simulink model "PID_robot_3d_base_movil"  (Simulink 7.5)
settings: Solver=ode45  StartTime=0.0  StopTime=50  RelTol=1e-3
libraries: simulink x3
settings Model: Creator=Patricio  LastModifiedBy=Patricio

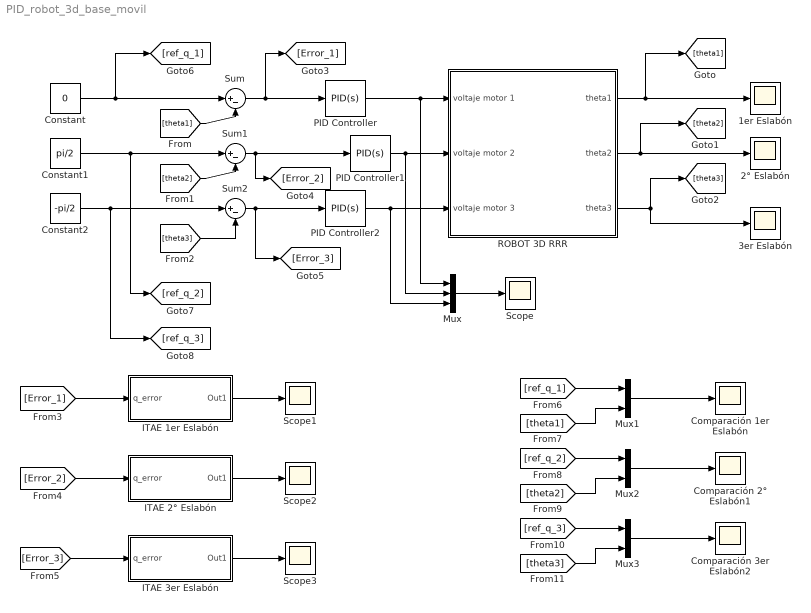
== system PID_robot_3d_base_movil ==
  1er Eslabón : Scope
      settings: TimeRange=5  YMin=-5000  YMax=-1750  MaxDataPoints=50000
  2° Eslabón : Scope
      settings: YMin=15.64  YMax=15.78  MaxDataPoints=50000
  3er Eslabón : Scope
      settings: TimeRange=30  YMin=-6.35  YMax=-6.21  SaveName=ScopeData2  MaxDataPoints=50000
  Comparación 1er Eslabón : Scope
      settings: TimeRange=30  YMin=-6.35  YMax=-6.21  SaveName=ScopeData10  MaxDataPoints=50000
  Comparación 2° Eslabón1 : Scope
      settings: TimeRange=30  YMin=-6.35  YMax=-6.21  SaveName=ScopeData8  MaxDataPoints=50000
  Comparación 3er Eslabón2 : Scope
      settings: TimeRange=30  YMin=-6.35  YMax=-6.21  SaveName=ScopeData18  MaxDataPoints=50000
  Constant : Constant  Value=0  OutDataType=fixdt(1, 16)  OutScaling=2^0
  Constant1 : Constant  Value=pi/2  OutDataType=fixdt(1, 16)  OutScaling=2^0
  Constant2 : Constant  Value=-pi/2  OutDataType=fixdt(1, 16)  OutScaling=2^0
  ITAE 1er Eslabón : Subsystem
  ITAE 2° Eslabón : Subsystem
  ITAE 3er Eslabón : Subsystem
  Mux : Mux  Inputs=3
  Mux1 : Mux  Inputs=2
  Mux2 : Mux  Inputs=2
  Mux3 : Mux  Inputs=2
  PID Controller : simulink/Continuous/PID Controller  DialogController=pidpack.PIDConfig.pidDDGCreate  DialogControllerArgs=DataTag0  SystemSampleTime=-1  Controller=PID  TimeDomain=Continuous-time  SampleTime=1  IntegratorMethod=Forward Euler  FilterMethod=Forward Euler  Form=Parallel  P=10  I=0  D=1  N=100  InitialConditionSource=internal  InitialConditionForIntegrator=0  InitialConditionForFilter=0  ExternalReset=none  LimitOutput=off  UpperSaturationLimit=inf  LowerSaturationLimit=-inf  LinearizeAsGain=off  AntiWindupMode=none  Kb=1  TrackingMode=off  Kt=1  PParamMin=[]  PParamMax=[]  IParamMin=[]  IParamMax=[]  DParamMin=[]  DParamMax=[]  NParamMin=[]  NParamMax=[]  KbParamMin=[]  KbParamMax=[]  KtParamMin=[]  KtParamMax=[]  POutMin=[]  POutMax=[]  IOutMin=[]  IOutMax=[]  DOutMin=[]  DOutMax=[]  NOutMin=[]  NOutMax=[]  KbOutMin=[]  KbOutMax=[]  KtOutMin=[]  KtOutMax=[]  IntegratorOutMin=[]  IntegratorOutMax=[]  FilterOutMin=[]  FilterOutMax=[]  SumOutMin=[]  SumOutMax=[]  SumI1OutMin=[]  SumI1OutMax=[]  SumI2OutMin=[]  SumI2OutMax=[]  SumI3OutMin=[]  SumI3OutMax=[]  SumDOutMin=[]  SumDOutMax=[]  SaturationOutMin=[]  SaturationOutMax=[]  IntegratorContinuousStateAttributes=''  IntegratorStateMustResolveToSignalObject=off  IntegratorRTWStateStorageClass=Auto  FilterContinuousStateAttributes=''  FilterStateMustResolveToSignalObject=off  FilterRTWStateStorageClass=Auto
  PID Controller1 : simulink/Continuous/PID Controller  DialogController=pidpack.PIDConfig.pidDDGCreate  DialogControllerArgs=DataTag1  SystemSampleTime=-1  Controller=PID  TimeDomain=Continuous-time  SampleTime=1  IntegratorMethod=Forward Euler  FilterMethod=Forward Euler  Form=Parallel  P=10  I=2  D=1  N=100  InitialConditionSource=internal  InitialConditionForIntegrator=0  InitialConditionForFilter=0  ExternalReset=none  LimitOutput=off  UpperSaturationLimit=inf  LowerSaturationLimit=-inf  LinearizeAsGain=off  AntiWindupMode=none  Kb=1  TrackingMode=off  Kt=1  PParamMin=[]  PParamMax=[]  IParamMin=[]  IParamMax=[]  DParamMin=[]  DParamMax=[]  NParamMin=[]  NParamMax=[]  KbParamMin=[]  KbParamMax=[]  KtParamMin=[]  KtParamMax=[]  POutMin=[]  POutMax=[]  IOutMin=[]  IOutMax=[]  DOutMin=[]  DOutMax=[]  NOutMin=[]  NOutMax=[]  KbOutMin=[]  KbOutMax=[]  KtOutMin=[]  KtOutMax=[]  IntegratorOutMin=[]  IntegratorOutMax=[]  FilterOutMin=[]  FilterOutMax=[]  SumOutMin=[]  SumOutMax=[]  SumI1OutMin=[]  SumI1OutMax=[]  SumI2OutMin=[]  SumI2OutMax=[]  SumI3OutMin=[]  SumI3OutMax=[]  SumDOutMin=[]  SumDOutMax=[]  SaturationOutMin=[]  SaturationOutMax=[]  IntegratorContinuousStateAttributes=''  IntegratorStateMustResolveToSignalObject=off  IntegratorRTWStateStorageClass=Auto  FilterContinuousStateAttributes=''  FilterStateMustResolveToSignalObject=off  FilterRTWStateStorageClass=Auto
  PID Controller2 : simulink/Continuous/PID Controller  DialogController=pidpack.PIDConfig.pidDDGCreate  DialogControllerArgs=DataTag2  SystemSampleTime=-1  Controller=PID  TimeDomain=Continuous-time  SampleTime=1  IntegratorMethod=Forward Euler  FilterMethod=Forward Euler  Form=Parallel  P=10  I=0  D=1  N=100  InitialConditionSource=internal  InitialConditionForIntegrator=0  InitialConditionForFilter=0  ExternalReset=none  LimitOutput=off  UpperSaturationLimit=inf  LowerSaturationLimit=-inf  LinearizeAsGain=off  AntiWindupMode=none  Kb=1  TrackingMode=off  Kt=1  PParamMin=[]  PParamMax=[]  IParamMin=[]  IParamMax=[]  DParamMin=[]  DParamMax=[]  NParamMin=[]  NParamMax=[]  KbParamMin=[]  KbParamMax=[]  KtParamMin=[]  KtParamMax=[]  POutMin=[]  POutMax=[]  IOutMin=[]  IOutMax=[]  DOutMin=[]  DOutMax=[]  NOutMin=[]  NOutMax=[]  KbOutMin=[]  KbOutMax=[]  KtOutMin=[]  KtOutMax=[]  IntegratorOutMin=[]  IntegratorOutMax=[]  FilterOutMin=[]  FilterOutMax=[]  SumOutMin=[]  SumOutMax=[]  SumI1OutMin=[]  SumI1OutMax=[]  SumI2OutMin=[]  SumI2OutMax=[]  SumI3OutMin=[]  SumI3OutMax=[]  SumDOutMin=[]  SumDOutMax=[]  SaturationOutMin=[]  SaturationOutMax=[]  IntegratorContinuousStateAttributes=''  IntegratorStateMustResolveToSignalObject=off  IntegratorRTWStateStorageClass=Auto  FilterContinuousStateAttributes=''  FilterStateMustResolveToSignalObject=off  FilterRTWStateStorageClass=Auto
  ROBOT 3D RRR : Subsystem
  Scope{,1..3} (4 alike) : Scope
      Scope settings: SaveName=ScopeData9
      Scope1 settings: SaveName=ScopeData15
      Scope2 settings: SaveName=ScopeData16
      Scope3 settings: SaveName=ScopeData17
  Sum : Sum  Inputs=|+-  OutDataType=fixdt(1, 16)  OutScaling=2^0
  Sum1 : Sum  Inputs=|+-  OutDataType=fixdt(1, 16)  OutScaling=2^0
  Sum2 : Sum  Inputs=|+-  OutDataType=fixdt(1, 16)  OutScaling=2^0
  wires:
  Sum/1 -> PID Controller/1, [Error_1]
  ROBOT 3D RRR/1(theta1) -> 1er Eslabón/1, [theta1]
  ROBOT 3D RRR/2(theta2) -> 2° Eslabón/1, [theta2]
  ROBOT 3D RRR/3(theta3) -> 3er Eslabón/1, [theta3]
  [theta1] -> Sum/2
  Sum1/1 -> PID Controller1/1, [Error_2]
  Sum2/1 -> PID Controller2/1, [Error_3]
  [theta2] -> Sum1/2
  [theta3] -> Sum2/2
  PID Controller/1 -> ROBOT 3D RRR/1(voltaje motor 1), Mux/1
  PID Controller1/1 -> ROBOT 3D RRR/2(voltaje motor 2), Mux/2
  PID Controller2/1 -> ROBOT 3D RRR/3(voltaje motor 3), Mux/3
  Mux/1 -> Scope/1
  Mux1/1 -> Comparación 1er Eslabón/1
  Constant2/1 -> Sum2/1, [ref_q_3]
  Constant1/1 -> Sum1/1, [ref_q_2]
  Constant/1 -> Sum/1, [ref_q_1]
  ITAE 1er Eslabón/1(Out1) -> Scope1/1
  ITAE 2° Eslabón/1(Out1) -> Scope2/1
  ITAE 3er Eslabón/1(Out1) -> Scope3/1
  [Error_1] -> ITAE 1er Eslabón/1(q_error)
  [Error_2] -> ITAE 2° Eslabón/1(q_error)
  [Error_3] -> ITAE 3er Eslabón/1(q_error)
  [ref_q_1] -> Mux1/1
  [theta1] -> Mux1/2
  Mux2/1 -> Comparación 2° Eslabón1/1
  [ref_q_2] -> Mux2/1
  [theta2] -> Mux2/2
  Mux3/1 -> Comparación 3er Eslabón2/1
  [ref_q_3] -> Mux3/1
  [theta3] -> Mux3/2

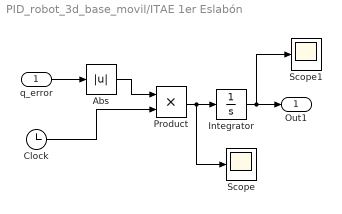
== system PID_robot_3d_base_movil/ITAE 1er Eslabón ==
  q_error : Inport  OutDataType=fixdt(1, 16)  OutScaling=2^0
  Abs : Abs  OutDataType=fixdt(1, 16)  OutScaling=2^0
  Clock : Clock
      settings: Decimation=10
  Integrator : Integrator
  Product : Product  OutDataType=fixdt(1, 16)  OutScaling=2^0  RndMeth=Zero
  Scope : Scope
      settings: SaveName=ScopeData6
  Scope1 : Scope
      settings: SaveName=ScopeData7
  Out1 : Outport  OutDataType=fixdt(1, 16)  OutScaling=2^0
  wires:
  q_error/1 -> Abs/1
  Abs/1 -> Product/1
  Clock/1 -> Product/2
  Product/1 -> Integrator/1, Scope/1
  Integrator/1 -> Out1/1, Scope1/1

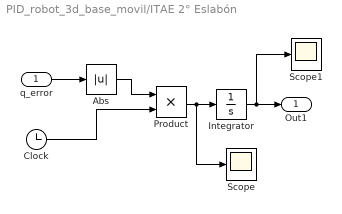
== system PID_robot_3d_base_movil/ITAE 2° Eslabón ==
  q_error : Inport  OutDataType=fixdt(1, 16)  OutScaling=2^0
  Abs : Abs  OutDataType=fixdt(1, 16)  OutScaling=2^0
  Clock : Clock
      settings: Decimation=10
  Integrator : Integrator
  Product : Product  OutDataType=fixdt(1, 16)  OutScaling=2^0  RndMeth=Zero
  Scope : Scope
      settings: SaveName=ScopeData6
  Scope1 : Scope
      settings: SaveName=ScopeData7
  Out1 : Outport  OutDataType=fixdt(1, 16)  OutScaling=2^0
  wires:
  Integrator/1 -> Scope1/1, Out1/1
  Product/1 -> Scope/1, Integrator/1
  Clock/1 -> Product/2
  Abs/1 -> Product/1
  q_error/1 -> Abs/1

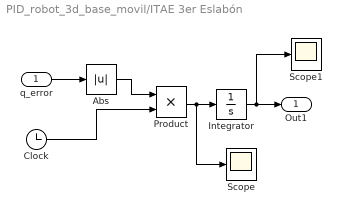
== system PID_robot_3d_base_movil/ITAE 3er Eslabón ==
  q_error : Inport  OutDataType=fixdt(1, 16)  OutScaling=2^0
  Abs : Abs  OutDataType=fixdt(1, 16)  OutScaling=2^0
  Clock : Clock
      settings: Decimation=10
  Integrator : Integrator
  Product : Product  OutDataType=fixdt(1, 16)  OutScaling=2^0  RndMeth=Zero
  Scope : Scope
      settings: SaveName=ScopeData6
  Scope1 : Scope
      settings: SaveName=ScopeData7
  Out1 : Outport  OutDataType=fixdt(1, 16)  OutScaling=2^0
  wires:
  q_error/1 -> Abs/1
  Abs/1 -> Product/1
  Clock/1 -> Product/2
  Product/1 -> Integrator/1, Scope/1
  Integrator/1 -> Out1/1, Scope1/1

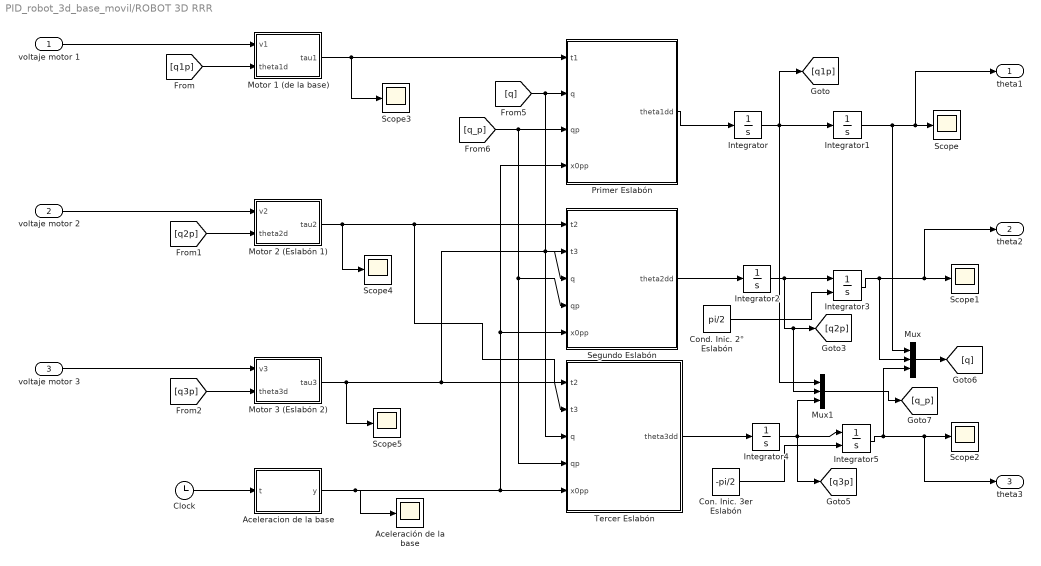
== system PID_robot_3d_base_movil/ROBOT 3D RRR ==
  voltaje motor 1 : Inport  OutDataType=fixdt(1, 16)  OutScaling=2^0
  voltaje motor 2 : Inport  Port=2  OutDataType=fixdt(1, 16)  OutScaling=2^0
  voltaje motor 3 : Inport  Port=3  OutDataType=fixdt(1, 16)  OutScaling=2^0
  Aceleracion de la base : Stateflow chart  TreatAsAtomicUnit=on
  Aceleración de la base : Scope
      settings: SaveName=ScopeData14  MaxDataPoints=50000
  Clock : Clock
      settings: Decimation=10
  Con. Inic. 3er Eslabón : Constant  Value=-pi/2  OutDataType=fixdt(1, 16)  OutScaling=2^0
  Cond. Inic. 2° Eslabón : Constant  Value=pi/2  OutDataType=fixdt(1, 16)  OutScaling=2^0
  Integrator{,1..2,4} (4 alike) : Integrator
  Integrator3 : Integrator  InitialConditionSource=external  InitialCondition=-pi/2
  Integrator5 : Integrator  InitialConditionSource=external
  Motor 1 (de la base) : Stateflow chart  TreatAsAtomicUnit=on
  Motor 2 (Eslabón 1) : Stateflow chart  TreatAsAtomicUnit=on
  Motor 3 (Eslabón 2) : Stateflow chart  TreatAsAtomicUnit=on
  Mux : Mux  Inputs=3
  Mux1 : Mux  Inputs=3
  Primer Eslabón : Stateflow chart  TreatAsAtomicUnit=on
      settings: MinAlgLoopOccurrences=on
  Scope{,1..5} (6 alike) : Scope
      Scope settings: SaveName=ScopeData3
      Scope1 settings: SaveName=ScopeData4
      Scope2 settings: SaveName=ScopeData5
      Scope3 settings: SaveName=ScopeData11
      Scope4 settings: SaveName=ScopeData12
      Scope5 settings: SaveName=ScopeData13
  Segundo Eslabón : Stateflow chart  TreatAsAtomicUnit=on
      settings: MinAlgLoopOccurrences=on
  Tercer Eslabón : Stateflow chart  TreatAsAtomicUnit=on
      settings: MinAlgLoopOccurrences=on
  theta1 : Outport  OutDataType=fixdt(1, 16)  OutScaling=2^0
  theta2 : Outport  Port=2  OutDataType=fixdt(1, 16)  OutScaling=2^0
  theta3 : Outport  Port=3  OutDataType=fixdt(1, 16)  OutScaling=2^0
  wires:
  Integrator/1 -> Integrator1/1, Mux1/1, [q1p]
  Primer Eslabón/1(theta1dd) -> Integrator/1
  Motor 1 (de la base)/1(tau1) -> Primer Eslabón/1(t1), Scope3/1
  [q] -> Primer Eslabón/2(q), Segundo Eslabón/3(q), Tercer Eslabón/3(q)
  [q_p] -> Primer Eslabón/3(qp), Segundo Eslabón/4(qp), Tercer Eslabón/4(qp)
  [q1p] -> Motor 1 (de la base)/2(theta1d)
  Motor 2 (Eslabón 1)/1(tau2) -> Scope4/1, Segundo Eslabón/1(t2), Tercer Eslabón/1(t2)
  [q2p] -> Motor 2 (Eslabón 1)/2(theta2d)
  Integrator2/1 -> Integrator3/1, [q2p], Mux1/2
  Integrator3/1 -> Mux/2, Scope1/1, theta2/1
  Motor 3 (Eslabón 2)/1(tau3) -> Scope5/1, Tercer Eslabón/2(t3), Segundo Eslabón/2(t3)
  Tercer Eslabón/1(theta3dd) -> Integrator4/1
  Integrator4/1 -> Integrator5/1, [q3p], Mux1/3
  Integrator5/1 -> Mux/3, Scope2/1, theta3/1
  [q3p] -> Motor 3 (Eslabón 2)/2(theta3d)
  Mux/1 -> [q]
  Mux1/1 -> [q_p]
  Segundo Eslabón/1(theta2dd) -> Integrator2/1
  Integrator1/1 -> Mux/1, Scope/1, theta1/1
  Cond. Inic. 2° Eslabón/1 -> Integrator3/2
  Con. Inic. 3er Eslabón/1 -> Integrator5/2
  Clock/1 -> Aceleracion de la base/1(t)
  Aceleracion de la base/1(y) -> Aceleración de la base/1, Tercer Eslabón/5(x0pp), Segundo Eslabón/5(x0pp), Primer Eslabón/4(x0pp)
  voltaje motor 3/1 -> Motor 3 (Eslabón 2)/1(v3)
  voltaje motor 2/1 -> Motor 2 (Eslabón 1)/1(v2)
  voltaje motor 1/1 -> Motor 1 (de la base)/1(v1)

== matlab function ROBOT 3D RRR/Aceleracion de la base ==
  data: t input double; y output double
function y = fcn(t)
%#eml
if t>=0 && t<2
    y=0;
elseif t>=2 && t<4
    y=0.5;
elseif t>=4 && t<6
    y=0;
elseif t>=6 && t<8
    y=-0.5;
else
    y=0;
end

== matlab function ROBOT 3D RRR/Motor 1 (de la base) ==
  data: v1 input double; tau1 output double; theta1d input double
function tau1 = fcn(v1,theta1d)
%#eml
%Voltaje entre 0 y 24 volts
N_1=50;
Kt=3; %en [volt/rad/seg]
Bm=0.1; %Roce viscozo [N.m/rad/seg]
R1=1;
tau1=(N_1*Kt*(v1/R1))-(Bm*theta1d);

== matlab function ROBOT 3D RRR/Primer Eslabón ==
  data: t1 input double; theta1dd output double; q input double size=3; qp input double size=3; x0pp input double
function theta1dd = fcn(t1,q,qp,x0pp)

theta1=q(1);
theta2=q(2);
theta3=q(3);

theta1d=qp(1);
theta2d=qp(2);
theta3d=qp(3);

a1=0.2;
a2=1;
a3=1;
b1=0.01;
%b2=0.01;
%b3=0.01;
%g=9.81;
m1=0.2;
m2=1;
m3=1;


theta1dd = (6*t1 - 6*b1*theta1d + 6*a1*m1*x0pp*sin(theta1) + 6*a1*m2*x0pp*sin(theta1) + 6*a1*m3*x0pp*sin(theta1) + 3*a2*m2*x0pp*cos(theta2)*sin(theta1) + 6*a2*m3*x0pp*cos(theta2)*sin(theta1) + 4*a2^2*m2*theta1d*theta2d*cos(theta2)*sin(theta2) + 12*a2^2*m3*theta1d*theta2d*cos(theta2)*sin(theta2) - 4*a3^2*m3*theta1d*theta2d*cos(theta2)*sin(theta2) - 4*a3^2*m3*theta1d*theta3d*cos(theta2)*sin(theta2) - 4*a3^2*m3*theta1d*theta2d*cos(theta3)*sin(theta3) - 4*a3^2*m3*theta1d*theta3d*cos(theta3)*sin(theta3) + 3*a3*m3*x0pp*cos(theta2)*cos(theta3)*sin(theta1) - 3*a3*m3*x0pp*sin(theta1)*sin(theta2)*sin(theta3) + 6*a1*a2*m2*theta1d*theta2d*sin(theta2) + 12*a1*a2*m3*theta1d*theta2d*sin(theta2) - 6*a2*a3*m3*theta1d*theta2d*sin(theta3) + 6*a1*a3*m3*theta1d*theta2d*cos(theta2)*sin(theta3) + 6*a1*a3*m3*theta1d*theta2d*cos(theta3)*sin(theta2) + 6*a1*a3*m3*theta1d*theta3d*cos(theta2)*sin(theta3) + 6*a1*a3*m3*theta1d*theta3d*cos(theta3)*sin(theta2) + 8*a3^2*m3*theta1d*theta2d*cos(theta2)*cos(theta3)^2*sin(theta2) + 8*a3^2*m3*theta1d*theta2d*cos(theta2)^2*cos(theta3)*sin(theta3) + 8*a3^2*m3*theta1d*theta3d*cos(theta2)*cos(theta3)^2*sin(theta2) + 8*a3^2*m3*theta1d*theta3d*cos(theta2)^2*cos(theta3)*sin(theta3) + 12*a2*a3*m3*theta1d*theta2d*cos(theta2)^2*sin(theta3) + 6*a2*a3*m3*theta1d*theta3d*cos(theta2)^2*sin(theta3) + 12*a2*a3*m3*theta1d*theta2d*cos(theta2)*cos(theta3)*sin(theta2) + 6*a2*a3*m3*theta1d*theta3d*cos(theta2)*cos(theta3)*sin(theta2))/(6*a1^2*m1 + 6*a1^2*m2 + 6*a1^2*m3 + 2*a3^2*m3 + 2*a2^2*m2*cos(theta2)^2 + 6*a2^2*m3*cos(theta2)^2 - 2*a3^2*m3*cos(theta2)^2 - 2*a3^2*m3*cos(theta3)^2 + 6*a1*a2*m2*cos(theta2) + 12*a1*a2*m3*cos(theta2) + 4*a3^2*m3*cos(theta2)^2*cos(theta3)^2 + 6*a1*a3*m3*cos(theta2)*cos(theta3) - 6*a1*a3*m3*sin(theta2)*sin(theta3) + 6*a2*a3*m3*cos(theta2)^2*cos(theta3) - 4*a3^2*m3*cos(theta2)*cos(theta3)*sin(theta2)*sin(theta3) - 6*a2*a3*m3*cos(theta2)*sin(theta2)*sin(theta3));

== matlab function ROBOT 3D RRR/Segundo Eslabón ==
  data: t2 input double; t3 input double; theta2dd output double; q input double size=3; qp input double size=3; x0pp input double
function theta2dd = fcn(t2,t3,q,qp,x0pp)

theta1=q(1);
theta2=q(2);
theta3=q(3);

theta1d=qp(1);
theta2d=qp(2);
theta3d=qp(3);

a1=0.2;
a2=1;
a3=1;
%b1=0.01;
b2=0.01;
b3=0.01;
g=9.81;
%m1=0.2;
m2=1;
m3=1;

theta2dd = (12*a3*t2 - 12*a3*t3 - 18*a2*t3*cos(theta3) - 12*a3*b2*theta2d + 12*a3*b3*theta3d + 18*a2*b3*theta3d*cos(theta3) + 6*a2*a3^2*m3*theta1d^2*sin(theta3) + 6*a2*a3^2*m3*theta2d^2*sin(theta3) + 6*a2*a3^2*m3*theta3d^2*sin(theta3) - 6*a2*a3*g*m2*cos(theta2) - 12*a2*a3*g*m3*cos(theta2) + 9*a2*a3*g*m3*cos(theta2)*cos(theta3)^2 - 4*a2^2*a3*m2*theta1d^2*cos(theta2)*sin(theta2) - 12*a2^2*a3*m3*theta1d^2*cos(theta2)*sin(theta2) + 9*a2^2*a3*m3*theta2d^2*cos(theta3)*sin(theta3) - 6*a1*a2*a3*m2*theta1d^2*sin(theta2) - 12*a1*a2*a3*m3*theta1d^2*sin(theta2) + 12*a2*a3^2*m3*theta2d*theta3d*sin(theta3) + 6*a2*a3*m2*x0pp*cos(theta1)*sin(theta2) + 12*a2*a3*m3*x0pp*cos(theta1)*sin(theta2) - 6*a2*a3^2*m3*theta1d^2*cos(theta2)^2*sin(theta3) - 6*a2*a3^2*m3*theta1d^2*cos(theta3)^2*sin(theta3) + 12*a2*a3^2*m3*theta1d^2*cos(theta2)^2*cos(theta3)^2*sin(theta3) - 12*a2*a3^2*m3*theta1d^2*cos(theta2)*cos(theta3)*sin(theta2) - 9*a2*a3*g*m3*cos(theta3)*sin(theta2)*sin(theta3) + 9*a2^2*a3*m3*theta1d^2*cos(theta2)*cos(theta3)^2*sin(theta2) + 12*a2*a3^2*m3*theta1d^2*cos(theta2)*cos(theta3)^3*sin(theta2) + 9*a2^2*a3*m3*theta1d^2*cos(theta2)^2*cos(theta3)*sin(theta3) + 9*a1*a2*a3*m3*theta1d^2*cos(theta3)^2*sin(theta2) - 9*a2*a3*m3*x0pp*cos(theta1)*cos(theta3)^2*sin(theta2) + 9*a1*a2*a3*m3*theta1d^2*cos(theta2)*cos(theta3)*sin(theta3) - 9*a2*a3*m3*x0pp*cos(theta1)*cos(theta2)*cos(theta3)*sin(theta3))/(4*a2^2*a3*m2 + 12*a2^2*a3*m3 - 9*a2^2*a3*m3*cos(theta3)^2);

== matlab function ROBOT 3D RRR/Motor 2 (Eslabón 1) ==
  data: v2 input double; tau2 output double; theta2d input double
function tau2 = fcn(v2,theta2d)
%#eml
%Voltaje entre 0 y 24 volts
N_1=50;
Kt=3; %en [volt/rad/seg]
Bm=0.1; %Roce viscozo [N.m/rad/seg]
R2=1;
tau2=(N_1*Kt*(v2/R2))-(Bm*theta2d);

== matlab function ROBOT 3D RRR/Motor 3 (Eslabón 2) ==
  data: v3 input double; tau3 output double; theta3d input double
function tau3 = fcn(v3,theta3d)
%#eml
%Voltaje entre 0 y 24 volts
N_1=50;
Kt=3; %en [volt/rad/seg]
Bm=0.1; %Roce viscozo [N.m/rad/seg]
R3=1;
tau3=(N_1*Kt*(v3/R3))-(Bm*theta3d);

== matlab function ROBOT 3D RRR/Tercer Eslabón ==
  data: t2 input double; t3 input double; theta3dd output double; q input double size=3; qp input double; x0pp input double
function theta3dd = fcn(t2,t3,q,qp,x0pp)

theta1=q(1);
theta2=q(2);
theta3=q(3);

theta1d=qp(1);
theta2d=qp(2);
theta3d=qp(3);

a1=0.2;
a2=1;
a3=1;
%b1=0.01;
b2=0.01;
b3=0.01;
g=9.81;
%m1=0.2;
m2=1;
m3=1;

theta3dd =-(12*a3^2*m3*t2 - 36*a2^2*m3*t3 - 12*a2^2*m2*t3 - 12*a3^2*m3*t3 + 12*a2^2*b3*m2*theta3d - 12*a3^2*b2*m3*theta2d + 36*a2^2*b3*m3*theta3d + 12*a3^2*b3*m3*theta3d + 6*a2*a3^3*m3^2*theta1d^2*sin(theta3) + 6*a2*a3^3*m3^2*theta2d^2*sin(theta3) + 18*a2^3*a3*m3^2*theta2d^2*sin(theta3) + 6*a2*a3^3*m3^2*theta3d^2*sin(theta3) - 12*a2*a3^2*g*m3^2*cos(theta2) + 18*a2*a3*m3*t2*cos(theta3) - 36*a2*a3*m3*t3*cos(theta3) + 6*a2^3*a3*m2*m3*theta2d^2*sin(theta3) + 12*a2*a3^3*m3^2*theta2d*theta3d*sin(theta3) - 18*a2*a3*b2*m3*theta2d*cos(theta3) + 36*a2*a3*b3*m3*theta3d*cos(theta3) - 24*a2^2*a3^2*m3^2*theta1d^2*cos(theta2)*sin(theta2) - 6*a2*a3^3*m3^2*theta1d^2*cos(theta2)^2*sin(theta3) - 3*a2^2*a3^2*m3^2*theta1d^2*cos(theta3)*sin(theta3) + 18*a2^3*a3*m3^2*theta1d^2*cos(theta2)^2*sin(theta3) - 6*a2*a3^3*m3^2*theta1d^2*cos(theta3)^2*sin(theta3) + 18*a2^2*a3^2*m3^2*theta2d^2*cos(theta3)*sin(theta3) + 9*a2^2*a3^2*m3^2*theta3d^2*cos(theta3)*sin(theta3) - 12*a1*a2*a3^2*m3^2*theta1d^2*sin(theta2) - 18*a2^2*a3*g*m3^2*sin(theta2)*sin(theta3) + 12*a2*a3^2*m3^2*x0pp*cos(theta1)*sin(theta2) - 6*a2*a3^2*g*m2*m3*cos(theta2) + 9*a2*a3^2*g*m3^2*cos(theta2)*cos(theta3)^2 + 12*a2*a3^3*m3^2*theta1d^2*cos(theta2)*cos(theta3)^3*sin(theta2) + 18*a1*a2^2*a3*m3^2*theta1d^2*cos(theta2)*sin(theta3) - 8*a2^2*a3^2*m2*m3*theta1d^2*cos(theta2)*sin(theta2) - 4*a2^2*a3^2*m2*m3*theta1d^2*cos(theta3)*sin(theta3) + 6*a2^3*a3*m2*m3*theta1d^2*cos(theta2)^2*sin(theta3) + 18*a2^2*a3^2*m3^2*theta2d*theta3d*cos(theta3)*sin(theta3) - 9*a2*a3^2*g*m3^2*cos(theta3)*sin(theta2)*sin(theta3) - 18*a2^2*a3*m3^2*x0pp*cos(theta1)*cos(theta2)*sin(theta3) - 3*a2^2*a3*g*m2*m3*cos(theta2)*cos(theta3) + 24*a2^2*a3^2*m3^2*theta1d^2*cos(theta2)*cos(theta3)^2*sin(theta2) + 24*a2^2*a3^2*m3^2*theta1d^2*cos(theta2)^2*cos(theta3)*sin(theta3) + 12*a2*a3^3*m3^2*theta1d^2*cos(theta2)^2*cos(theta3)^2*sin(theta3) - 6*a1*a2*a3^2*m2*m3*theta1d^2*sin(theta2) - 6*a2^2*a3*g*m2*m3*sin(theta2)*sin(theta3) + 6*a2*a3^2*m2*m3*x0pp*cos(theta1)*sin(theta2) + 9*a1*a2*a3^2*m3^2*theta1d^2*cos(theta3)^2*sin(theta2) - 12*a2*a3^3*m3^2*theta1d^2*cos(theta2)*cos(theta3)*sin(theta2) - 9*a2*a3^2*m3^2*x0pp*cos(theta1)*cos(theta3)^2*sin(theta2) + 9*a1*a2*a3^2*m3^2*theta1d^2*cos(theta2)*cos(theta3)*sin(theta3) - 9*a2*a3^2*m3^2*x0pp*cos(theta1)*cos(theta2)*cos(theta3)*sin(theta3) + 6*a1*a2^2*a3*m2*m3*theta1d^2*cos(theta2)*sin(theta3) - 3*a1*a2^2*a3*m2*m3*theta1d^2*cos(theta3)*sin(theta2) - 6*a2^2*a3*m2*m3*x0pp*cos(theta1)*cos(theta2)*sin(theta3) + 3*a2^2*a3*m2*m3*x0pp*cos(theta1)*cos(theta3)*sin(theta2) + 8*a2^2*a3^2*m2*m3*theta1d^2*cos(theta2)*cos(theta3)^2*sin(theta2) + 8*a2^2*a3^2*m2*m3*theta1d^2*cos(theta2)^2*cos(theta3)*sin(theta3))/(- 9*a2^2*a3^2*m3^2*cos(theta3)^2 + 12*a2^2*a3^2*m3^2 + 4*m2*a2^2*a3^2*m3);
